simulink model "pid_ecbf_sim"  (R2021a)
settings: Solver=VariableStepAuto  StartTime=0.0  StopTime=10.0  RelTol=1e-3
PreLoadFcn:
  | acc = [0 0 0]
undefined symbols (not defined in the file or in its folder): obstacle_trajectory, P, pid_controller, trajectory
settings Model: Creator=USER  LastModifiedBy=USER

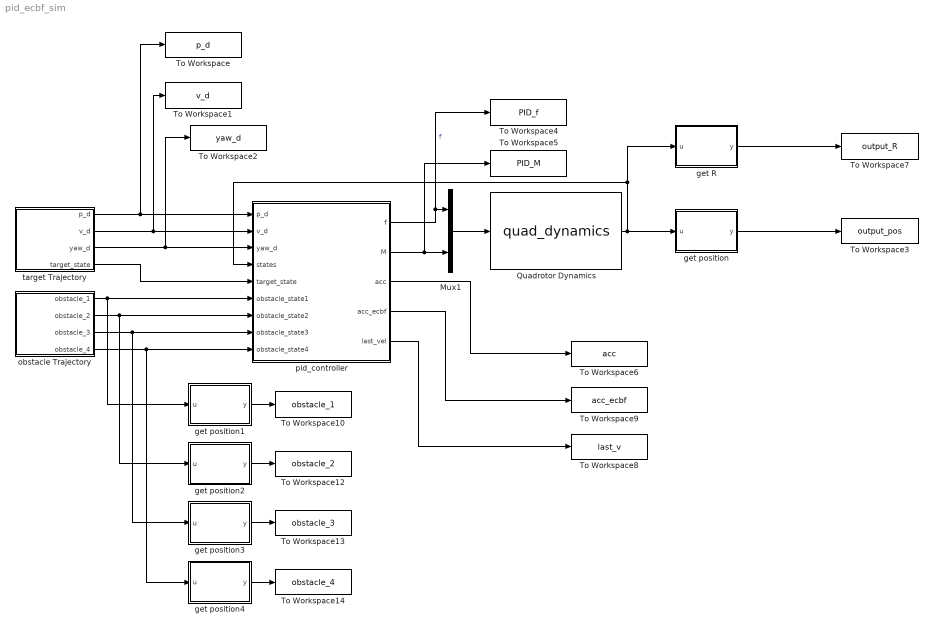
== system pid_ecbf_sim ==
  Mux1 : Mux  Inputs=2
  Quadrotor Dynamics : S-Function  FunctionName=quad_dynamics  Parameters=P  SFunctionDeploymentMode=off  EnableBusSupport=off
  To Workspace : ToWorkspace  VariableName=p_d  SaveFormat=Timeseries  SampleTime=-1
  To Workspace1 : ToWorkspace  VariableName=v_d  SaveFormat=Timeseries  SampleTime=-1
  To Workspace10 : ToWorkspace  VariableName=obstacle_1  SaveFormat=Timeseries  SampleTime=-1
  To Workspace12 : ToWorkspace  VariableName=obstacle_2  SaveFormat=Timeseries  SampleTime=-1
  To Workspace13 : ToWorkspace  VariableName=obstacle_3  SaveFormat=Timeseries  SampleTime=-1
  To Workspace14 : ToWorkspace  VariableName=obstacle_4  SaveFormat=Timeseries  SampleTime=-1
  To Workspace2 : ToWorkspace  VariableName=yaw_d  SaveFormat=Timeseries  SampleTime=-1
  To Workspace3 : ToWorkspace  VariableName=output_pos  SaveFormat=Timeseries  SampleTime=-1
  To Workspace4 : ToWorkspace  VariableName=PID_f  SaveFormat=Timeseries  SampleTime=-1
  To Workspace5 : ToWorkspace  VariableName=PID_M  SaveFormat=Timeseries  SampleTime=-1
  To Workspace6 : ToWorkspace  VariableName=acc  SaveFormat=Timeseries  SampleTime=-1
  To Workspace7 : ToWorkspace  VariableName=output_R  SaveFormat=Timeseries  SampleTime=-1
  To Workspace8 : ToWorkspace  VariableName=last_v  SaveFormat=Timeseries  SampleTime=-1
  To Workspace9 : ToWorkspace  VariableName=acc_ecbf  SaveFormat=Timeseries  SampleTime=-1
  get R : MATLAB Function  TreatAsAtomicUnit=on
  get position : MATLAB Function  TreatAsAtomicUnit=on
  get position1 : MATLAB Function  TreatAsAtomicUnit=on
  get position2 : MATLAB Function  TreatAsAtomicUnit=on
  get position3 : MATLAB Function  TreatAsAtomicUnit=on
  get position4 : MATLAB Function  TreatAsAtomicUnit=on
  obstacle Trajectory : Subsystem
  pid_controller : Subsystem
  target Trajectory : Subsystem
  wires:
  pid_controller/5(last_vel) -> To Workspace8/1
  target Trajectory/1(p_d) -> To Workspace/1, pid_controller/1(p_d)
  target Trajectory/3(yaw_d) -> To Workspace2/1, pid_controller/3(yaw_d)
  get R/1(y) -> To Workspace7/1
  pid_controller/2(M) -> To Workspace5/1, Mux1/2
  get position/1(y) -> To Workspace3/1
  pid_controller/1(f) -> To Workspace4/1, Mux1/1  "f"
  pid_controller/3(acc) -> To Workspace6/1
  Quadrotor Dynamics/1 -> get position/1(u), get R/1(u), pid_controller/4(states)
  Mux1/1 -> Quadrotor Dynamics/1
  target Trajectory/2(v_d) -> To Workspace1/1, pid_controller/2(v_d)
  target Trajectory/4(target_state) -> pid_controller/5(target_state)
  obstacle Trajectory/1(obstacle_1) -> get position1/1(u), pid_controller/6(obstacle_state1)
  obstacle Trajectory/2(obstacle_2) -> get position2/1(u), pid_controller/7(obstacle_state2)
  obstacle Trajectory/3(obstacle_3) -> get position3/1(u), pid_controller/8(obstacle_state3)
  pid_controller/4(acc_ecbf) -> To Workspace9/1
  get position1/1(y) -> To Workspace10/1
  get position2/1(y) -> To Workspace12/1
  get position4/1(y) -> To Workspace14/1
  get position3/1(y) -> To Workspace13/1
  obstacle Trajectory/4(obstacle_4) -> get position4/1(u), pid_controller/9(obstacle_state4)

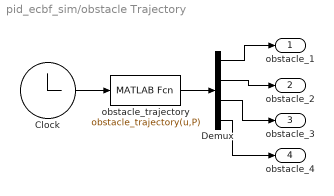
== system pid_ecbf_sim/obstacle Trajectory ==
  Clock : Clock
  Demux : Demux
  obstacle_trajectory : MATLABFcn  MATLABFcn=obstacle_trajectory(u,P)  OutputDimensions=40  SampleTime=P.Ts
  obstacle_1 : Outport  PortDimensions=10  VectorParamsAs1DForOutWhenUnconnected=off
  obstacle_2 : Outport  Port=2  PortDimensions=10  VectorParamsAs1DForOutWhenUnconnected=off
  obstacle_3 : Outport  Port=3  PortDimensions=10  VectorParamsAs1DForOutWhenUnconnected=off
  obstacle_4 : Outport  Port=4  PortDimensions=10  VectorParamsAs1DForOutWhenUnconnected=off
  wires:
  Demux/1 -> obstacle_1/1
  Demux/3 -> obstacle_3/1
  Demux/2 -> obstacle_2/1
  Clock/1 -> obstacle_trajectory/1
  obstacle_trajectory/1 -> Demux/1
  Demux/4 -> obstacle_4/1

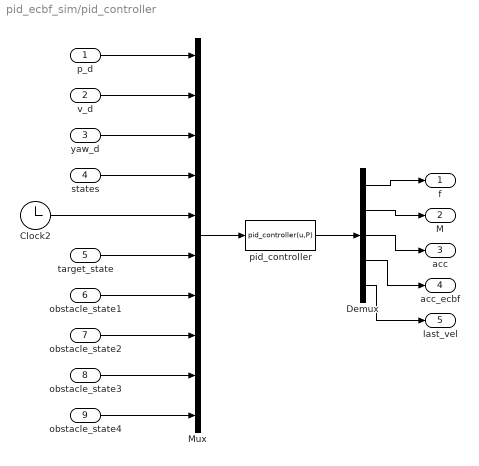
== system pid_ecbf_sim/pid_controller ==
  p_d : Inport
  v_d : Inport  Port=2
  yaw_d : Inport  Port=3
  states : Inport  Port=4
  target_state : Inport  Port=5
  obstacle_state1 : Inport  Port=6
  obstacle_state2 : Inport  Port=7
  obstacle_state3 : Inport  Port=8
  obstacle_state4 : Inport  Port=9
  Clock2 : Clock
  Demux : Demux  Outputs=5
  Mux : Mux  Inputs=10
  pid_controller : MATLABFcn  MATLABFcn=pid_controller(u,P)  OutputDimensions=13  SampleTime=P.Ts
  f : Outport  PortDimensions=1  VectorParamsAs1DForOutWhenUnconnected=off
  M : Outport  Port=2  PortDimensions=3  VectorParamsAs1DForOutWhenUnconnected=off
  acc : Outport  Port=3  PortDimensions=3  VectorParamsAs1DForOutWhenUnconnected=off
  acc_ecbf : Outport  Port=4  PortDimensions=3  VectorParamsAs1DForOutWhenUnconnected=off
  last_vel : Outport  Port=5  PortDimensions=3  VectorParamsAs1DForOutWhenUnconnected=off
  wires:
  p_d/1 -> Mux/1
  Demux/1 -> f/1
  Demux/2 -> M/1
  states/1 -> Mux/4
  Clock2/1 -> Mux/5
  yaw_d/1 -> Mux/3
  v_d/1 -> Mux/2
  Mux/1 -> pid_controller/1
  pid_controller/1 -> Demux/1
  Demux/3 -> acc/1
  Demux/5 -> last_vel/1
  target_state/1 -> Mux/6
  obstacle_state1/1 -> Mux/7
  obstacle_state2/1 -> Mux/8
  obstacle_state4/1 -> Mux/10
  obstacle_state3/1 -> Mux/9
  Demux/4 -> acc_ecbf/1

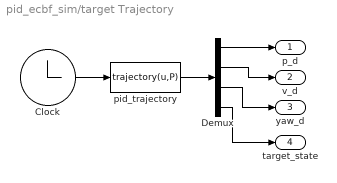
== system pid_ecbf_sim/target Trajectory ==
  Clock : Clock
  Demux : Demux
  pid_trajectory : MATLABFcn  MATLABFcn=trajectory(u,P)  OutputDimensions=17  SampleTime=P.Ts
  p_d : Outport  PortDimensions=3  VectorParamsAs1DForOutWhenUnconnected=off
  v_d : Outport  Port=2  PortDimensions=3  VectorParamsAs1DForOutWhenUnconnected=off
  yaw_d : Outport  Port=3  PortDimensions=1  VectorParamsAs1DForOutWhenUnconnected=off
  target_state : Outport  Port=4  PortDimensions=10  VectorParamsAs1DForOutWhenUnconnected=off
  wires:
  Demux/1 -> p_d/1
  Demux/3 -> yaw_d/1
  Demux/2 -> v_d/1
  Clock/1 -> pid_trajectory/1
  pid_trajectory/1 -> Demux/1
  Demux/4 -> target_state/1

== matlab function pid_ecbf_sim/get position1 ==
  data: u input; y output
function y = fcn(u)

y = u(1:3);

== matlab function pid_ecbf_sim/get R ==
  data: u input; y output
function y = fcn(u)

y = reshape(u(7:15),3,3);

== matlab function pid_ecbf_sim/get position2 ==
  data: u input; y output
function y = fcn(u)

y = u(1:3);

== matlab function pid_ecbf_sim/get position3 ==
  data: u input; y output
function y = fcn(u)

y = u(1:3);

== matlab function pid_ecbf_sim/get position4 ==
  data: u input; y output
function y = fcn(u)

y = u(1:3);

== matlab function pid_ecbf_sim/get position ==
  data: u input; y output
function y = fcn(u)

y = u(1:3);
